simulink model "controller"  (R2022b)
settings: Solver=VariableStepAuto  StartTime=0.0  StopTime=10.0  RelTol=1e-3
libraries: battery_monitor_lib x1, driver_interface_lib x1, governor_lib x1, motor_interface_lib x1, vehicle_dynamics_lib x1
settings Model: Creator=dr_pa  LastModifiedBy=dr_pa

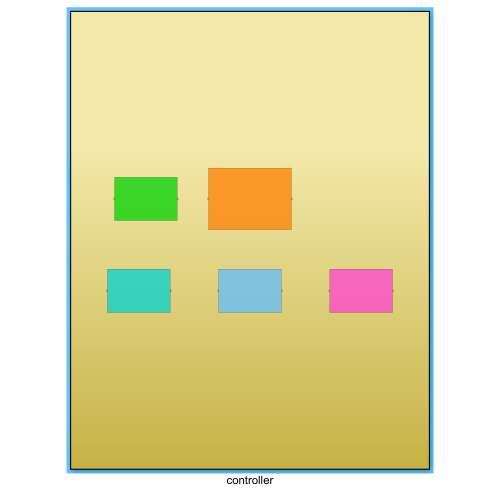
[thumbnail: Simulink's stored preview of the top-level diagram]
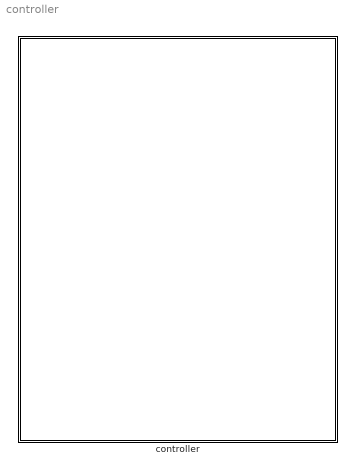
== system controller ==
  controller : Subsystem

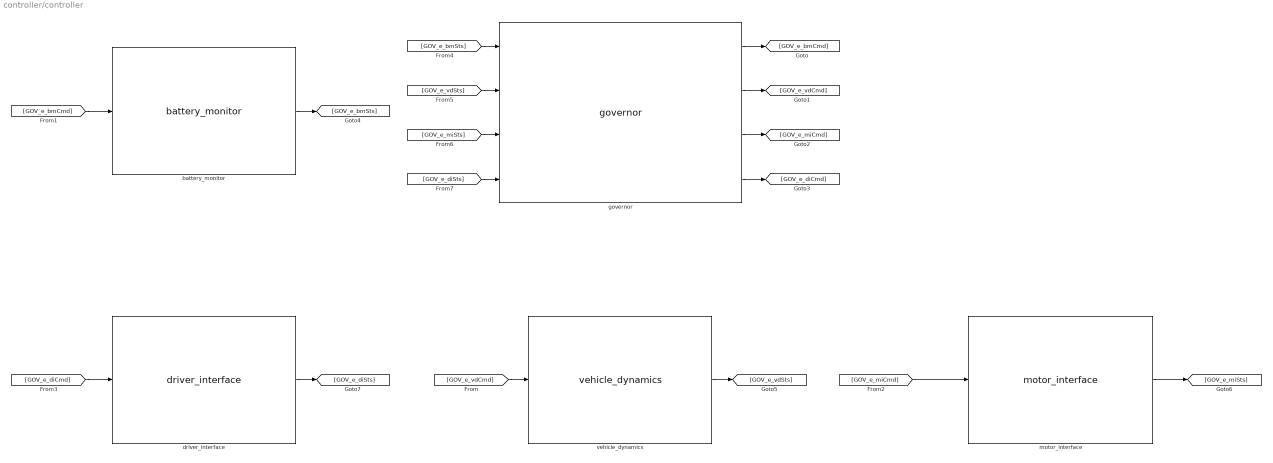
== system controller/controller ==
  battery_monitor : battery_monitor_lib/battery_monitor  SystemSampleTime=-1  VariantActivationTime=update diagram  Latency=0  AutoFrameSizeCalculation=off
  driver_interface : driver_interface_lib/driver_interface  SystemSampleTime=-1  VariantActivationTime=update diagram  Latency=0  AutoFrameSizeCalculation=off
  governor : governor_lib/governor  SystemSampleTime=-1  VariantActivationTime=update diagram  Latency=0  AutoFrameSizeCalculation=off
  motor_interface : motor_interface_lib/motor_interface  SystemSampleTime=-1  VariantActivationTime=update diagram  Latency=0  AutoFrameSizeCalculation=off
  vehicle_dynamics : vehicle_dynamics_lib/vehicle_dynamics  SystemSampleTime=-1  VariantActivationTime=update diagram  Latency=0  AutoFrameSizeCalculation=off
  wires:
  governor/1 -> [GOV_e_bmCmd]
  [GOV_e_bmCmd] -> battery_monitor/1
  [GOV_e_vdCmd] -> vehicle_dynamics/1
  governor/2 -> [GOV_e_vdCmd]
  governor/3 -> [GOV_e_miCmd]
  [GOV_e_miCmd] -> motor_interface/1
  governor/4 -> [GOV_e_diCmd]
  [GOV_e_diCmd] -> driver_interface/1
  battery_monitor/1 -> [GOV_e_bmSts]
  [GOV_e_bmSts] -> governor/1
  vehicle_dynamics/1 -> [GOV_e_vdSts]
  [GOV_e_vdSts] -> governor/2
  motor_interface/1 -> [GOV_e_miSts]
  [GOV_e_miSts] -> governor/3
  [GOV_e_diSts] -> governor/4
  driver_interface/1 -> [GOV_e_diSts]
